simulink model "Step_control"  (Simulink 8.0)
settings: Solver=ode45  StartTime=0.0  StopTime=10.0  RelTol=1e-3
settings Model: Creator=Faradars  LastModifiedBy=Faradars

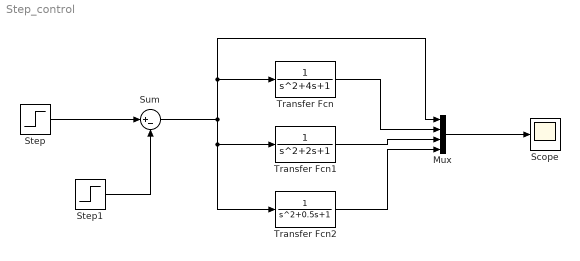
== system Step_control ==
  Mux : Mux
  Scope : Scope
  Step : Step  SampleTime=0
  Step1 : Step  Time=1.001  SampleTime=0
  Sum : Sum  Inputs=|+-
  Transfer Fcn : TransferFcn  Denominator=[1 4 1]
  Transfer Fcn1 : TransferFcn
  Transfer Fcn2 : TransferFcn  Denominator=[1 0.5 1]
  wires:
  Transfer Fcn/1 -> Mux/2
  Transfer Fcn1/1 -> Mux/3
  Transfer Fcn2/1 -> Mux/4
  Mux/1 -> Scope/1
  Step1/1 -> Sum/2
  Step/1 -> Sum/1
  Sum/1 -> Transfer Fcn/1, Mux/1, Transfer Fcn2/1, Transfer Fcn1/1
